simulink model "fc_dyn_c_sim"  (R2020b)
settings: Solver=FixedStepAuto  StartTime=0.0  StopTime=tend  FixedStep=dt  RelTol=1e-3
values from neighbouring files (symbols this model uses):
  dt = 0.01    [input_sine.m]    (also in input_step.m)
  Rsys = 0.1^2    (= 0.01)    [input_sine.m]    (also in input_step.m)
  x0 = [0.21;0.21;1;1;1]    [OptGain.m]    (also in input_sine.m = [xch_O2c;xch_O2c;J_ss;J_ss;J_ss]; input_step.m = [xch_O2c;xch_O2c;J_ss;J_ss;J_ss])
undefined symbols (not defined in the file or in its folder): param
settings Model: Creator=kvijayar  LastModifiedBy=kvijayar

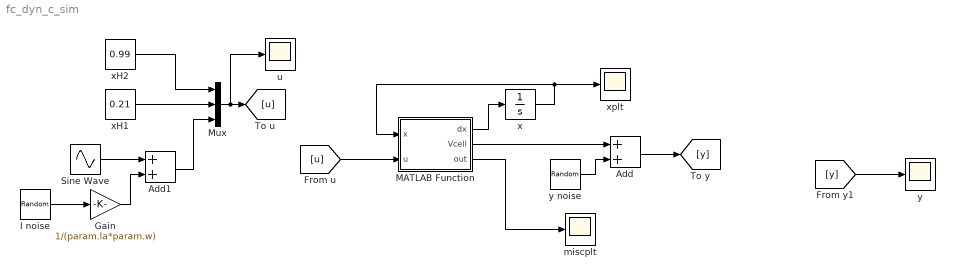
== system fc_dyn_c_sim ==
  Add : Sum
  Add1 : Sum
  Gain : Gain  Gain=1/(param.la*param.w)
  I noise : RandomNumber  Variance=Rsys  SampleTime=dt
  MATLAB Function : MATLAB Function  TreatAsAtomicUnit=on
  Mux : Mux  Inputs=3
  Sine Wave : Sin  Amplitude=5000  Bias=5000  Phase=-pi/2  SampleTime=0
  miscplt : Scope
  u : Scope
  x : Integrator  InitialCondition=x0
  xH1 : Constant  Value=0.21
  xH2 : Constant  Value=0.99
  xplt : Scope
  y : Scope
  y noise : RandomNumber  Variance=Rsys  SampleTime=dt
  wires:
  Add/1 -> [y]
  x/1 -> xplt/1, MATLAB Function/1(x)
  y noise/1 -> Add/2
  Add1/1 -> Mux/3
  I noise/1 -> Gain/1
  xH2/1 -> Mux/1
  [u] -> MATLAB Function/2(u)
  MATLAB Function/2(Vcell) -> Add/1
  MATLAB Function/1(dx) -> x/1
  Gain/1 -> Add1/2
  MATLAB Function/3(out) -> miscplt/1
  xH1/1 -> Mux/2
  [y] -> y/1
  Sine Wave/1 -> Add1/1
  Mux/1 -> u/1, [u]

== matlab function fc_dyn_c_sim/MATLAB Function ==
  data: dx output; x input; u input; Vcell output; param parameter; out output; dt parameter
function [dx,Vcell,out] = F(x,u,param,dt)

Vcell = 0;
flag_start = 8; flag_dyn = 4; flag_dyn_starve = 4+2;

% if dt == 0; flag = flag_start; else; flag = flag_dyn_starve; end
flag = flag_dyn;
Area = (param.la*param.w);

coder.extrinsic('fc_dyn_c'); % Declare 'fc_dyn_c' as extrinsic so the MEX file can run
% Originally: [V, xH2a, xO2c, xH2c, T_tmp, J, JR, Jhf, xO2hf, xO2hf1 ] = fc_dyn_c(I, param, flag, dt);
[V, xH2a, xO2c, xH2c, ~, ~] = fc_dyn_c(u(3)*Area, param, flag, dt);
dx = 0;
out=0;
Vcell = V;
